simulink model "Pratica6Analise"  (R2020a)
settings: Solver=VariableStepAuto  StartTime=0.0  StopTime=10  RelTol=1e-3
settings Model: Creator=laris  LastModifiedBy=laris

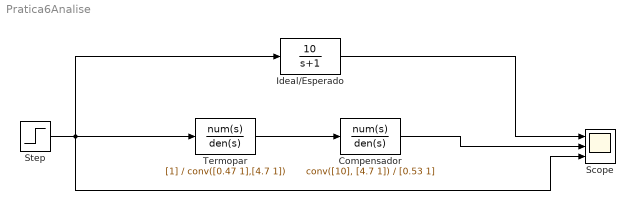
== system Pratica6Analise ==
  Compensador : TransferFcn  Numerator=conv([10], [4.7 1])  Denominator=[0.53 1]
  Ideal/Esperado : TransferFcn  Numerator=10  Denominator=[1 1]
  Scope : Scope  NumInputPorts=3
  Step : Step  Time=0  SampleTime=0
  Termopar : TransferFcn  Denominator=conv([0.47 1],[4.7 1])
  wires:
  Step/1 -> Ideal/Esperado/1, Scope/3, Termopar/1
  Termopar/1 -> Compensador/1
  Compensador/1 -> Scope/2
  Ideal/Esperado/1 -> Scope/1
